simulink model "Xmer_Susa_swift"  (R2020a)
settings: Solver=VariableStepAuto  StartTime=0.0  StopTime=500  RelTol=1e-3
InitFcn:
  | d1=1;
  | d2=1;
  | d3=3
  | d4=3;
  | d5 = 5;
  | d6 = 5;
  | Tau=9
libraries: simulink x2
settings Model: Creator=SHAAD  LastModifiedBy=Hozefa Jesawada
settings DataIOCC: ReturnWorkspaceOutputs=off
settings DebuggingCC: ArithmeticOperatorsInVariantConditions=warning
settings SFSimCC: SimUseLocalCustomCode=off  CustomCodeUndefinedFunction=UseInterfaceOnly
settings RTWCC: RTWUseLocalCustomCode=off
settings CodeAppCC: StateflowObjectComments=on

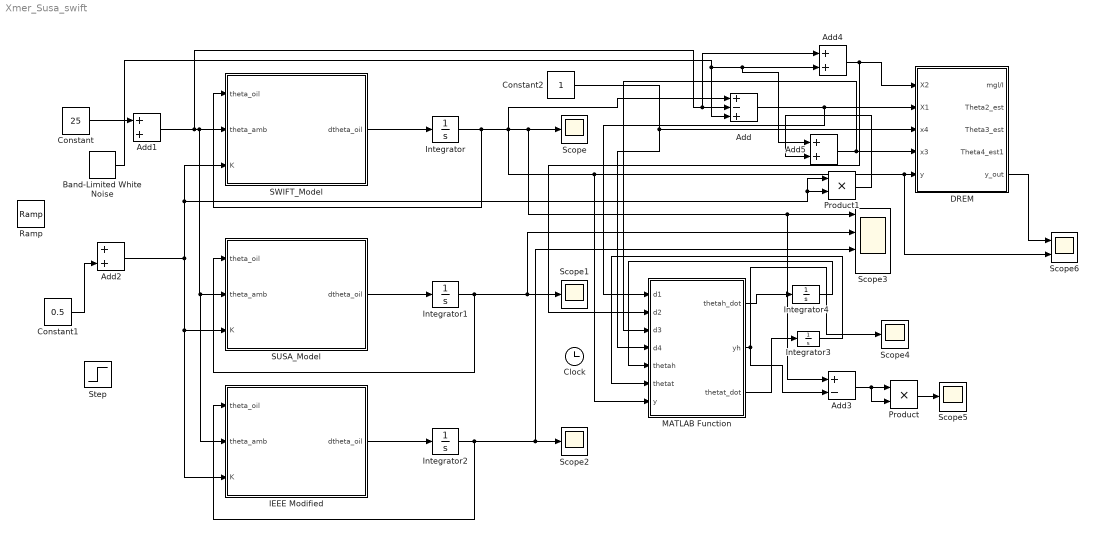
== system Xmer_Susa_swift ==
  Add : Sum  Inputs=+-+
  Add{1..2,4..5} (4 alike) : Sum
  Add3 : Sum  Inputs=+-
  Band-Limited White Noise : simulink/Sources/Band-Limited White Noise  Cov=[0.1]  Ts=0.1  seed=[23341]
  Clock : Clock
  Constant : Constant  Value=25
  Constant1 : Constant  Value=0.5
  Constant2 : Constant
  DREM : Subsystem
  IEEE Modified : MATLAB Function  TreatAsAtomicUnit=on
  Integrator : Integrator  InitialCondition=42
  Integrator1 : Integrator  InitialCondition=42
  Integrator2 : Integrator  InitialCondition=42
  Integrator3 : Integrator  InitialCondition=[0;0;0;0]
  Integrator4 : Integrator  InitialCondition=[0;0;0;0]
  MATLAB Function : MATLAB Function  TreatAsAtomicUnit=on
  Product : Product
  Product1 : Product
  Ramp : simulink/Sources/Ramp  slope=0.0001  start=0  InitialOutput=0
  SUSA_Model : MATLAB Function  TreatAsAtomicUnit=on
  SWIFT_Model : MATLAB Function  TreatAsAtomicUnit=on
  Scope{,1..2,4..5} (5 alike) : Scope
  Scope3 : Scope  NumInputPorts=4
  Scope6 : Scope  NumInputPorts=2
  Step : Step  SampleTime=0
  wires:
  SWIFT_Model/1(dtheta_oil) -> Integrator/1
  SUSA_Model/1(dtheta_oil) -> Integrator1/1
  Integrator1/1 -> Scope3/2, Scope1/1, SUSA_Model/1(theta_oil)
  IEEE Modified/1(dtheta_oil) -> Integrator2/1
  Integrator2/1 -> Scope3/3, Scope2/1, IEEE Modified/1(theta_oil)
  Integrator/1 -> Add/1, Scope6/2, DREM/5(y), MATLAB Function/7(y), Add3/1, Scope3/1, Scope/1, SWIFT_Model/1(theta_oil)
  Constant2/1 -> MATLAB Function/4(d4), DREM/3(x4)
  Add2/1 -> IEEE Modified/3(K), SUSA_Model/3(K), SWIFT_Model/3(K), Product1/2, Product1/1
  Band-Limited White Noise/1 -> Add5/1, Add4/2, Add/3
  Constant/1 -> Add1/1
  Add1/1 -> IEEE Modified/2(theta_amb), SUSA_Model/2(theta_amb), SWIFT_Model/2(theta_amb), Add4/1, Add/2
  Constant1/1 -> Add2/2
  MATLAB Function/3(thetat_dot) -> Integrator3/1
  MATLAB Function/1(thetah_dot) -> Integrator4/1
  MATLAB Function/2(yh) -> Scope4/1, Add3/2
  Integrator3/1 -> MATLAB Function/6(thetat)
  Integrator4/1 -> MATLAB Function/5(thetah)
  Add/1 -> MATLAB Function/1(d1), DREM/2(X1)
  Add3/1 -> Product/2, Product/1
  Product/1 -> Scope5/1
  DREM/5(y_out) -> Scope6/1
  Product1/1 -> Add5/2
  ? -> Add2/1
  Add4/1 -> MATLAB Function/2(d2), DREM/1(X2)
  Add5/1 -> MATLAB Function/3(d3), DREM/4(x3)

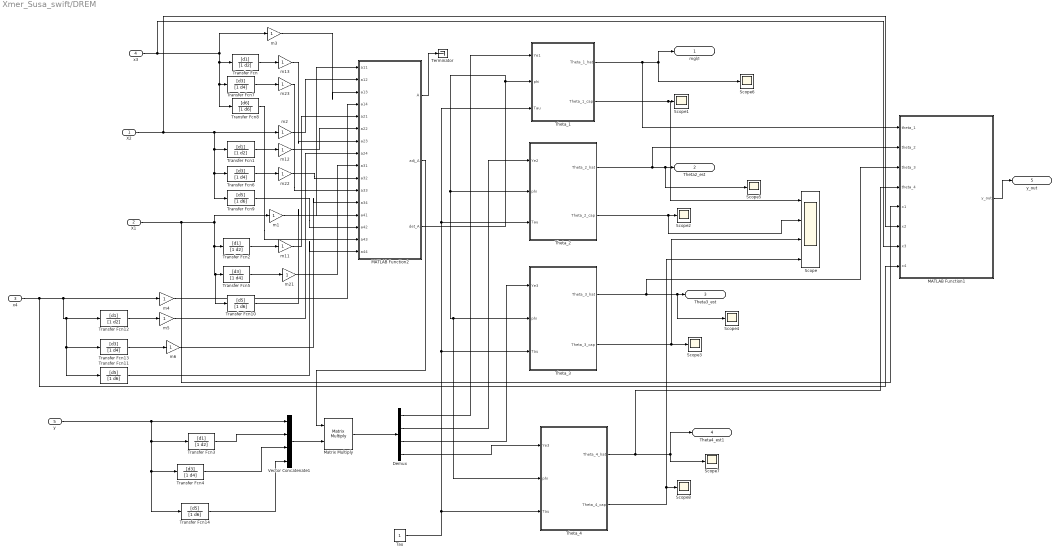
== system Xmer_Susa_swift/DREM ==
  X2 : Inport
  X1 : Inport  Port=2
  x4 : Inport  Port=3
  x3 : Inport  Port=4
  y : Inport  Port=5
  Demux : Demux
  MATLAB Function1 : MATLAB Function  TreatAsAtomicUnit=on
  MATLAB Function2 : MATLAB Function  TreatAsAtomicUnit=on
  Matrix Multiply : Product  Multiplication=Matrix(*)
  Scope : Scope  NumInputPorts=4
  Scope{1..8} (8 alike) : Scope
  Tau : Constant  SampleTime=-1
  Terminator : Terminator
  Theta_1 : Subsystem
  Theta_2 : Subsystem
  Theta_3 : Subsystem
  Theta_4 : Subsystem
  Transfer Fcn{,1..3,12} (5 alike) : TransferFcn  Numerator=[d1]  Denominator=[1 d2]
  Transfer Fcn{9..11,14} (4 alike) : TransferFcn  Numerator=[d5]  Denominator=[1 d6]
  Transfer Fcn{4..7,13} (5 alike) : TransferFcn  Numerator=[d3]  Denominator=[1 d4]
  Transfer Fcn8 : TransferFcn  Numerator=[d6]  Denominator=[1 d6]
  Vector Concatenate1 : Concatenate  NumInputs=4
  m{1..6,11..13,21..23} (12 alike) : Gain
  mgl/I : Outport
  Theta2_est : Outport  Port=2
  Theta3_est : Outport  Port=3
  Theta4_est1 : Outport  Port=4
  y_out : Outport  Port=5
  wires:
  Transfer Fcn/1 -> m13/1
  Transfer Fcn7/1 -> m23/1
  Transfer Fcn1/1 -> m12/1
  Transfer Fcn6/1 -> m22/1
  Transfer Fcn5/1 -> m21/1
  Transfer Fcn3/1 -> Vector Concatenate1/2
  y/1 -> Transfer Fcn14/1, Transfer Fcn4/1, Transfer Fcn3/1, Vector Concatenate1/1
  Transfer Fcn4/1 -> Vector Concatenate1/3
  MATLAB Function2/3(det_A) -> Theta_4/2(phi), Theta_3/2(phi), Theta_2/2(phi), Theta_1/2(phi)
  Tau/1 -> Theta_3/3(Tau), Theta_1/3(Tau), Theta_2/3(Tau), Theta_4/3(Tau)
  m1/1 -> MATLAB Function2/1(a11)
  m11/1 -> MATLAB Function2/5(a21)
  m21/1 -> MATLAB Function2/9(a31)
  m2/1 -> MATLAB Function2/2(a12)
  m12/1 -> MATLAB Function2/6(a22)
  m22/1 -> MATLAB Function2/10(a32)
  m3/1 -> MATLAB Function2/3(a13)
  m13/1 -> MATLAB Function2/7(a23)
  m23/1 -> MATLAB Function2/11(a33)
  Theta_1/1(Theta_1_hat) -> MATLAB Function1/1(theta_1), mgl/I/1, Scope6/1
  Theta_1/2(Theta_1_cap) -> Scope1/1, Scope/1
  Theta_2/1(Theta_2_hat) -> MATLAB Function1/2(theta_2), Scope5/1, Theta2_est/1
  Theta_2/2(Theta_2_cap) -> Scope/2, Scope2/1
  Theta_3/1(Theta_3_hat) -> MATLAB Function1/3(theta_3), Scope4/1, Theta3_est/1
  Theta_3/2(Theta_3_cap) -> Scope/3, Scope3/1
  Transfer Fcn2/1 -> m11/1
  Vector Concatenate1/1 -> Matrix Multiply/2
  MATLAB Function2/2(adj_A) -> Matrix Multiply/1
  Matrix Multiply/1 -> Demux/1
  Demux/1 -> Theta_1/1(Ye1)
  Demux/2 -> Theta_2/1(Ye2)
  Demux/3 -> Theta_3/1(Ye3)
  x3/1 -> MATLAB Function1/7(x3), m3/1, Transfer Fcn8/1, Transfer Fcn7/1, Transfer Fcn/1
  X2/1 -> MATLAB Function1/6(x2), Transfer Fcn9/1, Transfer Fcn6/1, Transfer Fcn1/1, m2/1
  Transfer Fcn10/1 -> MATLAB Function2/13(a41)
  Transfer Fcn11/1 -> MATLAB Function2/16(a44)
  m4/1 -> MATLAB Function2/4(a14)
  m6/1 -> MATLAB Function2/12(a34)
  Transfer Fcn12/1 -> m5/1
  x4/1 -> MATLAB Function1/8(x4), Transfer Fcn12/1, Transfer Fcn11/1, Transfer Fcn13/1, m4/1
  Transfer Fcn13/1 -> m6/1
  m5/1 -> MATLAB Function2/8(a24)
  Transfer Fcn8/1 -> MATLAB Function2/15(a43)
  Transfer Fcn9/1 -> MATLAB Function2/14(a42)
  Transfer Fcn14/1 -> Vector Concatenate1/4
  Demux/4 -> Theta_4/1(Ye3)
  MATLAB Function2/1(A) -> Terminator/1
  Theta_4/1(Theta_4_hat) -> MATLAB Function1/4(theta_4), Theta4_est1/1, Scope7/1
  Theta_4/2(Theta_4_cap) -> Scope/4, Scope8/1
  X1/1 -> MATLAB Function1/5(x1), m1/1, Transfer Fcn2/1, Transfer Fcn10/1, Transfer Fcn5/1
  MATLAB Function1/1(y_out) -> y_out/1

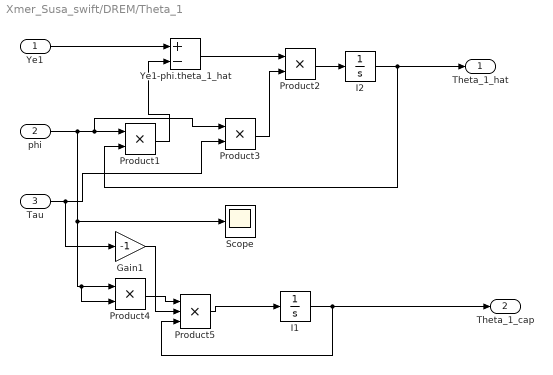
== system Xmer_Susa_swift/DREM/Theta_1 ==
  Ye1 : Inport
  phi : Inport  Port=2
  Tau : Inport  Port=3
  Gain1 : Gain  Gain=-1
  I1 : Integrator  InitialCondition=9.8
  I2 : Integrator
  Product{1..4} (4 alike) : Product
  Product5 : Product  Inputs=3
  Scope : Scope
  Ye1-phi.theta_1_hat : Sum  Inputs=+-
  Theta_1_hat : Outport
  Theta_1_cap : Outport  Port=2
  wires:
  Ye1/1 -> Ye1-phi.theta_1_hat/1
  phi/1 -> Scope/1, Product4/2, Product4/1, Product3/1, Product1/1
  Ye1-phi.theta_1_hat/1 -> Product2/1
  Product1/1 -> Ye1-phi.theta_1_hat/2
  Product3/1 -> Product2/2
  Tau/1 -> Gain1/1, Product3/2
  Product2/1 -> I2/1
  Product5/1 -> I1/1
  Product4/1 -> Product5/1
  Gain1/1 -> Product5/2
  I1/1 -> Product5/3, Theta_1_cap/1
  I2/1 -> Product1/2, Theta_1_hat/1

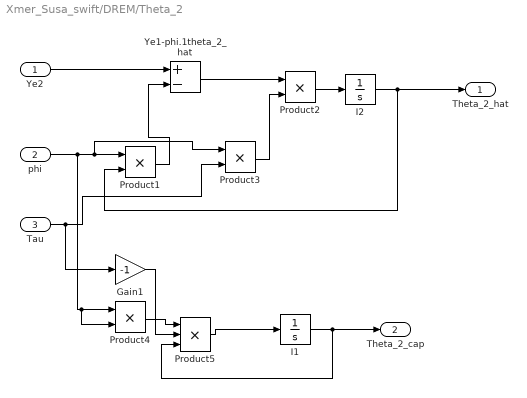
== system Xmer_Susa_swift/DREM/Theta_2 ==
  Ye2 : Inport
  phi : Inport  Port=2
  Tau : Inport  Port=3
  Gain1 : Gain  Gain=-1
  I1 : Integrator  InitialCondition=96.27
  I2 : Integrator
  Product{1..4} (4 alike) : Product
  Product5 : Product  Inputs=3
  Ye1-phi.1theta_2_hat : Sum  Inputs=+-
  Theta_2_hat : Outport
  Theta_2_cap : Outport  Port=2
  wires:
  Ye2/1 -> Ye1-phi.1theta_2_hat/1
  phi/1 -> Product4/2, Product4/1, Product3/1, Product1/1
  Ye1-phi.1theta_2_hat/1 -> Product2/1
  Product1/1 -> Ye1-phi.1theta_2_hat/2
  Product3/1 -> Product2/2
  Tau/1 -> Gain1/1, Product3/2
  Product2/1 -> I2/1
  Product5/1 -> I1/1
  Product4/1 -> Product5/1
  Gain1/1 -> Product5/2
  I1/1 -> Product5/3, Theta_2_cap/1
  I2/1 -> Product1/2, Theta_2_hat/1

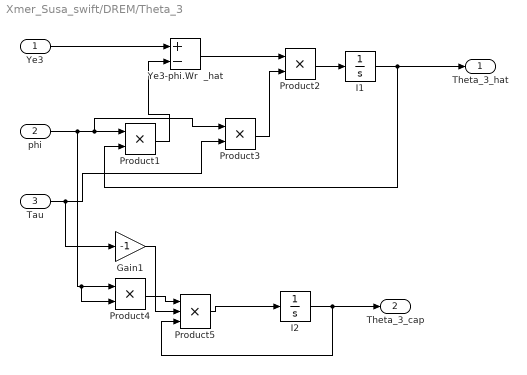
== system Xmer_Susa_swift/DREM/Theta_3 ==
  Ye3 : Inport
  phi : Inport  Port=2
  Tau : Inport  Port=3
  Gain1 : Gain  Gain=-1
  I1 : Integrator
  I2 : Integrator  InitialCondition=12000
  Product{1..4} (4 alike) : Product
  Product5 : Product  Inputs=3
  Ye3-phi.Wr  _hat : Sum  Inputs=+-
  Theta_3_hat : Outport
  Theta_3_cap : Outport  Port=2
  wires:
  Ye3/1 -> Ye3-phi.Wr  _hat/1
  phi/1 -> Product4/2, Product4/1, Product3/1, Product1/1
  Ye3-phi.Wr  _hat/1 -> Product2/1
  Product1/1 -> Ye3-phi.Wr  _hat/2
  Product3/1 -> Product2/2
  Tau/1 -> Gain1/1, Product3/2
  Product2/1 -> I1/1
  Product5/1 -> I2/1
  Product4/1 -> Product5/1
  Gain1/1 -> Product5/2
  I2/1 -> Product5/3, Theta_3_cap/1
  I1/1 -> Product1/2, Theta_3_hat/1

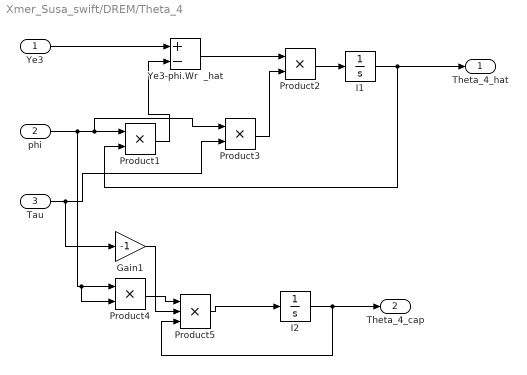
== system Xmer_Susa_swift/DREM/Theta_4 ==
  Ye3 : Inport
  phi : Inport  Port=2
  Tau : Inport  Port=3
  Gain1 : Gain  Gain=-1
  I1 : Integrator
  I2 : Integrator  InitialCondition=100
  Product{1..4} (4 alike) : Product
  Product5 : Product  Inputs=3
  Ye3-phi.Wr  _hat : Sum  Inputs=+-
  Theta_4_hat : Outport
  Theta_4_cap : Outport  Port=2
  wires:
  Ye3/1 -> Ye3-phi.Wr  _hat/1
  phi/1 -> Product4/2, Product4/1, Product3/1, Product1/1
  Ye3-phi.Wr  _hat/1 -> Product2/1
  Product1/1 -> Ye3-phi.Wr  _hat/2
  Product3/1 -> Product2/2
  Tau/1 -> Gain1/1, Product3/2
  Product2/1 -> I1/1
  Product5/1 -> I2/1
  Product4/1 -> Product5/1
  Gain1/1 -> Product5/2
  I2/1 -> Product5/3, Theta_4_cap/1
  I1/1 -> Product1/2, Theta_4_hat/1

== matlab function Xmer_Susa_swift/SUSA_Model ==
  data: theta_oil input; dtheta_oil output; theta_amb input; K input
function dtheta_oil = fcn(theta_oil, theta_amb, K)
%Parameters
Del_theta_oilR=48;
R=6;
n=0.8;
tau_oilR=150;
theta_oilR=70;
%theta_amb=35;
%K=0.85;
A=1.3573e-6*exp((2797.3)/(theta_oil+273));
B=1.3573e-6*exp((2797.3)/(theta_oilR+273));
a=(1-n)/n;
mu_pu=A/B;
dtheta_oil =(((Del_theta_oilR))/tau_oilR)*[(K*K*R+1)/(R+1)]-(1/tau_oilR)*[((theta_oil-theta_amb)^(1/n))/(mu_pu*theta_oilR)^a];

== matlab function Xmer_Susa_swift/SWIFT_Model ==
  data: theta_oil input; dtheta_oil output; theta_amb input; K input
function dtheta_oil = fcn(theta_oil, theta_amb, K)
%Parameters
Del_theta_oilR=48;
R=6;
n=0.75;
tau_oilR=200;
%theta_amb=35;
%K=0.85;
dtheta_oil =(((Del_theta_oilR)^(1/n))/tau_oilR)*[(K*K*R+1)/(R+1)]-(1/tau_oilR)*[theta_oil-theta_amb]^(1/n) ;

== matlab function Xmer_Susa_swift/IEEE Modified ==
  data: theta_oil input; dtheta_oil output; theta_amb input; K input
function dtheta_oil = fcn(theta_oil, theta_amb, K)
%Parameters
Del_theta_oilR=48;
R=6;
n=0.8;
tau_oilR=150;
%theta_amb=35;
%K=0.85;
dtheta_oil =(((Del_theta_oilR))/tau_oilR)*[(K*K*R+1)/(R+1)]^n+(1/tau_oilR)*[theta_amb-theta_oil] ;

== matlab function Xmer_Susa_swift/DREM/MATLAB Function2 ==
  data: a11 input; a12 input; a13 input; a14 input; a21 input; A output; a22 input; a23 input; a24 input; a31 input; a32 input; a33 input; a34 input; a41 input; a42 input; a43 input; a44 input; adj_A output; det_A output
function [A,adj_A,det_A]  = MATRIX(a11,a12,a13,a14,a21,a22,a23,a24,a31,a32,a33,a34,a41,a42,a43,a44)
A = [a11,a12,a13,a14;a21,a22,a23,a24;a31,a32,a33,a34;a41,a42,a43,a44];     
[m,n]=size(A);
if m ~= n, return, end
AD = ones(m);
for ki=1:n
   for kj = 1:n
      AD(ki,kj) = (-1)^(ki+kj)*det(A([1:ki-1 ki+1:n],[1:kj-1 kj+1:n]));
   end
end
adj_A =AD';
det_A = det(A);

end

== matlab function Xmer_Susa_swift/DREM/MATLAB Function1 ==
  data: theta_1 input; theta_2 input; theta_3 input; theta_4 input; x1 input; y_out output; x2 input; x3 input; x4 input
function y_out  = MATRIX(theta_1,theta_2,theta_3,theta_4,x1,x2,x3,x4)
m = [theta_1;theta_2;theta_3;theta_4];
X=[x1;x2;x3;x4];
y_out=m'*X;
end

== matlab function Xmer_Susa_swift/MATLAB Function ==
  data: d1 input; d2 input; d3 input; d4 input; thetah_dot output; yh output; thetat_dot output; thetah input; thetat input; y input
function [thetah_dot, yh,  thetat_dot]= fcn(d1,d2,d3,d4, thetah, thetat,y)
M=[d1; d2; d3; d4 ];%Regressor
theta=[1;1;1;1];%Parameter
%y = M'*theta;
tau=1000;
thetah_dot=tau*M*(y-M'*thetah);%gradient Estimator
thetat_dot=-tau*M*M'*thetat;
yh=M'*thetah;
